simulink model "ControlDesignOnrampwithSimulink_Task1"  (R2022b)
settings: Solver=VariableStepAuto  StartTime=0.0  StopTime=5  RelTol=1e-3
StartFcn:
  | learning.simulink.modelCallbacks.startFunction(gcs)
StopFcn:
  | learning.simulink.modelCallbacks.stopFunction(gcs);
model workspace (MAT data in the model file):
  courseObject.course = 'controls'
  courseObject.chapter = 6
  courseObject.lesson = 1
  courseObject.section = 3
  courseObject.task = 1
  t_ans = [0; 1.8; 1.8; 1.8; 1.8; 5]
  y_ans = [0; 0; 0; 0; 0; 0; 0; 0; 0; 0; 0; 0; 0.698325580681; 2.45203860716; 4.61534825253; 6.54855382994; 7.8016035065; 8.20611579525; 7.86788923154; 7.082576098; 6.21390760403; 5.57620090878; 5.35376643717; 5.57333048024; 6.12725885651; 6.83099976725; 7.49141181018; 7.9640661338; 8.18518697067; 8.17412128684; 8.01151317106; 7.80422962664; 7.64964970064; 7.60964888049; 7.69984883547; 7.89424983039; 8.14091081114; 8.38200045613; 8.57159343777; 8.68654569166; 8.72869713874; 8.7194827888; 8.68998913037; 8.67019486556; 8.68063504357; 8.72840194768; 8.80778067619; 8.90442990031; 9.00121390691; 9.08368960226; 9.14374369156; 9.18070176974]
  y_ans_lower = [0; 0; 0; 0; 9.7; 9.7]
  y_ans_upper = [11.1; 11.1; 11.1; 11.1; 10.3; 10.3]
undefined symbols (not defined in the file): g, Kd, L, m
libraries: slpidlib x1
CloseFcn:
  | learning.simulink.cleanupOnlineTraining
Description:
  | Training model
settings Model: Creator=AhmedSamy  LastModifiedBy=AhmedSamy
settings DataIOCC: SaveTime=off

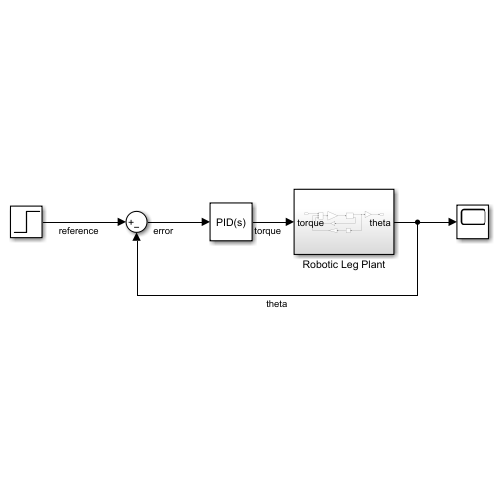
[thumbnail: Simulink's stored preview of the top-level diagram]
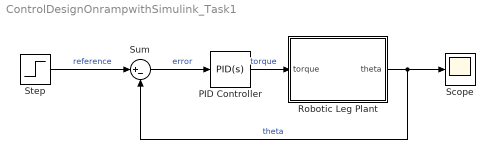
== system ControlDesignOnrampwithSimulink_Task1 ==
  PID Controller : slpidlib/PID Controller  Controller=PID  Form=Parallel  TimeDomain=Continuous-time  UseExternalTs=off  SampleTime=-1  IntegratorMethod=Forward Euler  FilterMethod=Forward Euler  ControllerParametersSource=internal  P=35.3138034695258  I=87.4594565789379  UseKiTs=off  D=3.55342604525185  N=6239.02802503553  UseFilter=on  TunerSelectOption=Transfer Function Based (PID Tuner App)  InitialConditionSource=internal  InitialConditionForIntegrator=0  InitialConditionForFilter=0  DifferentiatorICPrevScaledInput=0  ExternalReset=none  TrackingMode=off  Kt=1  LimitOutput=off  SatLimitsSource=internal  UpperSaturationLimit=inf  LowerSaturationLimit=-inf  LinearizeAsGain=on  AntiWindupMode=none  Kb=1  LimitIntegrator=off  UpperIntegratorSaturationLimit=inf  LowerIntegratorSaturationLimit=-inf  POutMin=[]  POutMax=[]  IOutMin=[]  IOutMax=[]  DOutMin=[]  DOutMax=[]  NOutMin=[]  NOutMax=[]  SumOutMin=[]  SumOutMax=[]  SaturationOutMin=[]  SaturationOutMax=[]  PParamMin=[]  PParamMax=[]  IParamMin=[]  IParamMax=[]  DParamMin=[]  DParamMax=[]  NParamMin=[]  NParamMax=[]  KbParamMin=[]  KbParamMax=[]  KtParamMin=[]  KtParamMax=[]  KbOutMin=[]  KbOutMax=[]  KtOutMin=[]  KtOutMax=[]  IntegratorOutMin=[]  IntegratorOutMax=[]  FilterOutMin=[]  FilterOutMax=[]  SumI1OutMin=[]  SumI1OutMax=[]  SumI2OutMin=[]  SumI2OutMax=[]  SumI3OutMin=[]  SumI3OutMax=[]  SumI4OutMin=[]  SumI4OutMax=[]  SumDOutMin=[]  SumDOutMax=[]  DifferentiatorOutMin=[]  DifferentiatorOutMax=[]  FilterDiffOutCoefMin=[]  FilterDiffOutCoefMax=[]  ReciprocalOutMin=[]  ReciprocalOutMax=[]  SumDenOutMin=[]  SumDenOutMax=[]  SumNumOutMin=[]  SumNumOutMax=[]  DivideOutMin=[]  DivideOutMax=[]  UdiffTsProdOutMin=[]  UdiffTsProdOutMax=[]  NTsProdOutMin=[]  NTsProdOutMax=[]  UintegralTsProdOutMin=[]  UintegralTsProdOutMax=[]  UngainTsProdOutMin=[]  UngainTsProdOutMax=[]  ClampingZeroOutDataTypeStr=Inherit: Inherit via back propagation  ClampingZeroOutMin=[]  ClampingZeroOutMax=[]  FilterDenConstantOutDataTypeStr=Inherit: Inherit via back propagation  FilterDenConstantOutMin=[]  FilterDenConstantOutMax=[]  PCopyOutDataTypeStr=Inherit: Inherit via back propagation  PCopyOutMin=[]  PCopyOutMax=[]  NCopyOutDataTypeStr=Inherit: Inherit via back propagation  NCopyOutMin=[]  NCopyOutMax=[]  IntegratorContinuousStateAttributes=''  IntegratorStateMustResolveToSignalObject=off  IntegratorRTWStateStorageClass=Auto  FilterContinuousStateAttributes=''  FilterStateMustResolveToSignalObject=off  FilterRTWStateStorageClass=Auto  ParallelPVariant=InternalParameters  IdealPVariant=Disabled  IVariant=InternalParameters  DVariant=InternalParameters  IntegratorVariant=Continuous  SatVariant=Disabled  AWVariant=Passthrough  PCopyVariant=Disabled  TRVariant=Disabled  FdbkBlocksVariant=Forward  IdealPFdbkVariant=Disabled  SatFdbkVariant=Disabled  DerivativeFilterVariant=ContFilter  NVariant=InternalParameters  NCopyVariant=Disabled  FilterICVariant=InternalICsFilter  IntegratorICVariant=InternalICs  ExternalResetVariant=Disabled  TRSumVariant=Passthrough  SumFdbkVariant=Disabled  SumVariant=Sum_PID  TsampFilterVariant=InternalTs  TsampNgainVariant=Passthrough  TsampIntegralVariant=Passthrough  ExternalSaturationOutDataTypeStr=Inherit: Same as second input
  Robotic Leg Plant : Subsystem
  Scope : Scope
  Step : Step  After=10  SampleTime=0
  Sum : Sum  Inputs=|+-
  wires:
  Robotic Leg Plant/1(theta) -> Scope/1, Sum/2  "theta"
  PID Controller/1 -> Robotic Leg Plant/1(torque)  "torque"
  Sum/1 -> PID Controller/1  "error"
  Step/1 -> Sum/1  "reference"

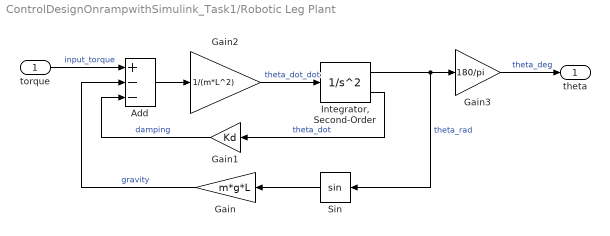
== system ControlDesignOnrampwithSimulink_Task1/Robotic Leg Plant ==
  torque : Inport
  Add : Sum  Inputs=+--
  Gain : Gain  Gain=m*g*L
  Gain1 : Gain  Gain=Kd
  Gain2 : Gain  Gain=1/(m*L^2)
  Gain3 : Gain  Gain=180/pi
  "Integrator, Second-Order" : SecondOrderIntegrator  ICX=0  LimitX=on  UpperLimitX=pi/4  LowerLimitX=-pi/4
  Sin : Trigonometry
  theta : Outport
  wires:
  Gain3/1 -> theta/1  "theta_deg"
  Gain1/1 -> Add/3  "damping"
  Sin/1 -> Gain/1
  Gain/1 -> Add/2  "gravity"
  Gain2/1 -> "Integrator, Second-Order"/1  "theta_dot_dot"
  "Integrator, Second-Order"/1 -> Sin/1, Gain3/1  "theta_rad"
  "Integrator, Second-Order"/2 -> Gain1/1  "theta_dot"
  Add/1 -> Gain2/1
  torque/1 -> Add/1  "input_torque"
